simulink model "pll_now01"  (Simulink 8.1)
settings: Solver=ode45  StartTime=1  StopTime=4  MaxStep=0.000001  RelTol=1e-3
libraries: dsparch4 x2, commsynccomp2 x1, simulink x1
settings Model: Creator=my88899  LastModifiedBy=my88899
settings SolverCC: ConsecutiveZCsStepRelTol=20*128*eps
settings DataIOCC: SignalLoggingSaveFormat=Dataset
settings OptimizationCC: ExpressionDepthLimit=128
settings DebuggingCC: FcnCallInpInsideContextMsg=EnableAllAsError
settings GRTTargetCC: CombineOutputUpdateFcns=on  GRTInterface=off

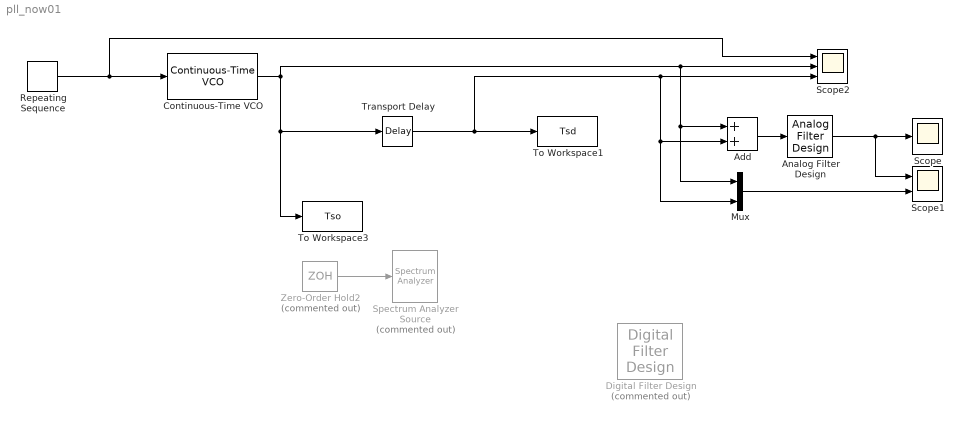
== system pll_now01 ==
  Add : Sum
  Analog Filter Design : dsparch4/Analog Filter Design  method=Butterworth  filttype=Lowpass  N=12  Wlo=2*3.14*40000  Whi=80  Rp=2  Rs=40
  Continuous-Time VCO : commsynccomp2/Continuous-Time VCO  Ac=5  Fc=10000  Kc=10000  Ph=0
  Digital Filter Design : dsparch4/Digital Filter Design  Commented=on  mwdsp_browser_bugfix_var=off
  Mux : Mux  Inputs=2
  Repeating Sequence : simulink/Sources/Repeating Sequence  rep_seq_t=[0 2]  rep_seq_y=[0 4]
  Scope : Scope
      settings: TimeRange=0.1038961038961048  YMin=-20  YMax=20  MaxDataPoints=10000001
  Scope1 : Scope  NumInputPorts=2
      settings: TimeRange=0.1038961038961048  YMin=-15~-15  YMax=15~15  MaxDataPoints=10000001
  Scope2 : Scope  NumInputPorts=3
      settings: TimeRange=0.1038961038961048  YMin=3.05~-5~-5  YMax=3.5~5~5  MaxDataPoints=100000
  "Spectrum Analyzer Source " : SpectrumAnalyzer  Commented=on
      settings: CopyFcn=scopeextensions.ScopeBlock.callback(gcbh, 'onBlockCopy', gcbh);  DeleteFcn=scopeextensions.ScopeBlock.callback(gcbh, 'onBlockDelete');  PreSaveFcn=scopeextensions.ScopeBlock.callback(gcbh, 'onModelSave');  NameChangeFcn=scopeextensions.ScopeBlock.callback(gcbh, 'onBlockRename');  CloseFcn=scopeextensions.ScopeBlock.callback(gcbh, 'onBlockClose');  PreDeleteFcn=scopeextensions.ScopeBlock.callback(gcbh, 'onBlockPreDelete');
  To Workspace1 : ToWorkspace  VariableName=Tsd  SampleTime=-1  SaveFormat=Timeseries
  To Workspace3 : ToWorkspace  VariableName=Tso  SampleTime=-1  SaveFormat=Timeseries
  Transport Delay : TransportDelay  DelayTime=0.3  BufferSize=200000
  Zero-Order Hold2 : ZeroOrderHold  Commented=on  SampleTime=0.001
  wires:
  Repeating Sequence/1 -> Scope2/1, Continuous-Time VCO/1
  Zero-Order Hold2/1 -> "Spectrum Analyzer Source "/1
  Continuous-Time VCO/1 -> To Workspace3/1, Transport Delay/1, Mux/1, Add/1, Scope2/2
  Transport Delay/1 -> Mux/2, Add/2, Scope2/3, To Workspace1/1
  Add/1 -> Analog Filter Design/1
  Mux/1 -> Scope1/2
  Analog Filter Design/1 -> Scope/1, Scope1/1
